simulink model "IM_Model"  (R2023a)
settings: Solver=ode23t  StartTime=0.0  StopTime=2  MaxStep=.0001  RelTol=1e-3
InitFcn:
  | Rs=0.5968;
  | Lls=0.0003495;
  | Rr=0.6258;
  | Llr=0.005473;
  | Lm=0.0354;
  | Ls=Lls+Lm;
  | Lr=Llr+Lm;
  | J=0.05;
  | B=0.005879;
  | P=4;
values from neighbouring files (symbols this model uses):
  Freq = 2*pi*50    (= 314.159265359)    [Parameters.m]
  Lms = Lm    (= 0.0353505)    [Parameters.m]
  Vin_Amp = 220*sqrt(2)    [Parameters.m]
libraries: spsControlledVoltageSourceLib x3, spsdq0toabcLib x2, spsAsynchronousMachineSIUnitsLib x1, spsabctodq0Lib x1, spspowerguiLib x1
settings Model: Creator=User  LastModifiedBy=User
settings DebuggingCC: UnconnectedInputMsg=warning  UnconnectedOutputMsg=warning  UnconnectedLineMsg=warning
settings ModelReferenceCC: EnableRefExpFcnMdlSchedulingChecks=on
settings RTWCC: DLArmComputeVersion=19.05

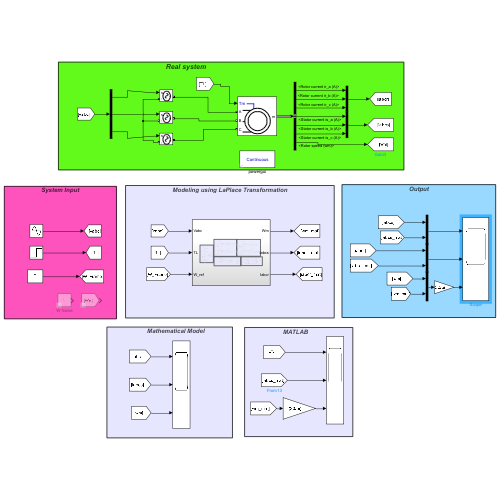
[thumbnail: Simulink's stored preview of the top-level diagram]
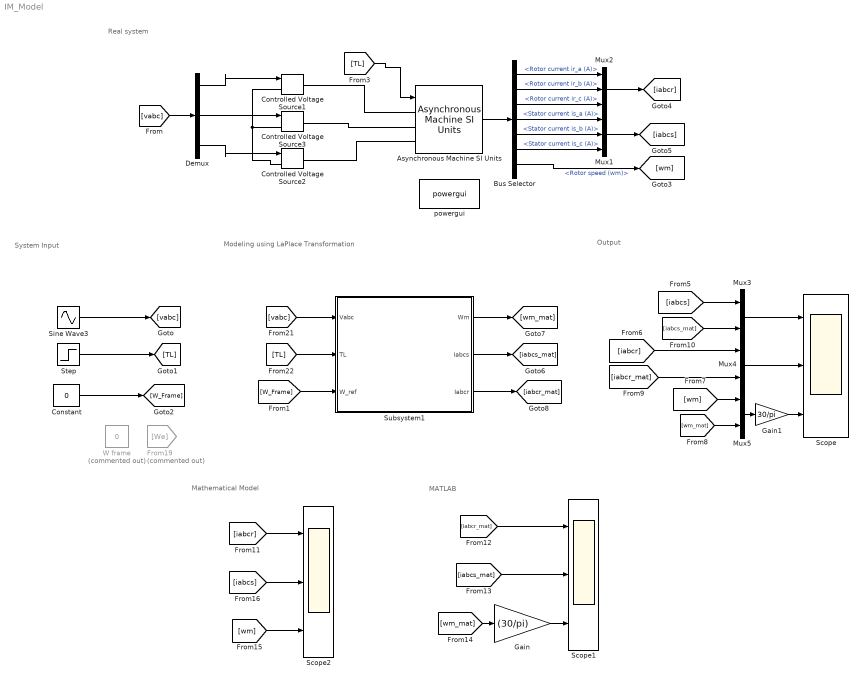
== system IM_Model ==
  note: Mathematical Model
  note: MATLAB
  note: Modeling using LaPlace Transformation
  note: Output
  note: System Input
  note: Real system
  Asynchronous Machine SI Units : spsAsynchronousMachineSIUnitsLib/Asynchronous Machine SI Units  RotorType=Squirrel-cage  PresetModel=No  MechanicalLoad=Torque Tm  ShowDetailedParameters=on  ReferenceFrame=Stationary  Units=SI  MeasurementBus=off  NominalParameters=[1e+04 400 50]  VoltageRatio=1  Stator=[Rs Lls]  Rotor=[Rr Llr]  Cage1=[0.4155 0.002066]  Cage2=[0.4168 0.0003495]  Lm=Lm  Mechanical=[J B P/2]  PolePairs=2  InitialConditions=[1 0 0 0 0 0 0 0]  SimulateSaturation=off  Saturation=[14.03593122, 27.81365428, 53.79336849, 72.68890987, 97.98006896, 148.6815601, 215.7428561, 302.9841135, 428.7778367 ; 230, 322, 414, 460, 506, 552, 598, 644, 690]  LoadFlowParameters=1492000  TsPowergui=0  TsBlock=-1  IterativeModel=Trapezoidal non iterative  IterativeDiscreteModel=Trapezoidal non iterative  Pmec=1.492e+006
  Bus Selector : BusSelector  OutputSignals=Rotor measurements.Rotor current ir_a (A),Rotor measurements.Rotor current ir_b (A),Rotor measurements.Rotor current ir_c (A),Stator measurements.Stator current is_a (A),Stator measurements.Stator current is_b (A),Stator measurements.Stator current is_c (A),Mechanical.Rotor speed (wm)
  Constant : Constant  Value=0
  Controlled Voltage Source1 : spsControlledVoltageSourceLib/Controlled Voltage Source  Initialize=on  Source_Type=AC  Amplitude=0  Phase=0  Frequency=0  Measurements=None
  Controlled Voltage Source2 : spsControlledVoltageSourceLib/Controlled Voltage Source  Initialize=on  Source_Type=AC  Amplitude=0  Phase=0  Frequency=0  Measurements=None
  Controlled Voltage Source3 : spsControlledVoltageSourceLib/Controlled Voltage Source  Initialize=on  Source_Type=AC  Amplitude=0  Phase=0  Frequency=0  Measurements=None
  Demux : Demux  Outputs=3
  From19 : From  Commented=on  GotoTag=We
  Gain : Gain  Gain=(30/pi)
  Gain1 : Gain  Gain=30/pi
  Mux1 : Mux  Inputs=3
  Mux2 : Mux  Inputs=3
  Mux3 : Mux  Inputs=2
  Mux4 : Mux  Inputs=2
  Mux5 : Mux  Inputs=2
  Scope : Scope  NumInputPorts=3
  Scope1 : Scope  NumInputPorts=3
  Scope2 : Scope  NumInputPorts=3
  Sine Wave3 : Sin  Amplitude=Vin_Amp  Frequency=Freq  Phase=[0 -2*pi/3 2*pi/3]  SampleTime=0
  Step : Step  Time=0  SampleTime=0
  Subsystem1 : Subsystem
  W frame : Constant  Commented=on  Value=0
  powergui : spspowerguiLib/powergui  Priority=1  SimulationMode=Continuous  SampleTime=50e-6  frequency=60  Iterations=50  frequencyindice=50  Pbase=100e6  ErrMax=1e-4  UnitsV=kV  UnitsW=MW  buscounter=0  FunctionMessages=off  echomessages=off  EnableUseOfTLC=off  CurrentSourceSwitches=off  DisableSnubberDevices=on  DisableRonSwitches=on  DisableVfSwitches=on  DisplayEquations=off  AutomaticDiscreteSolvers=off  SolverType=Tustin/Backward Euler (TBE)  Interpol=off  ExternalGateDelay=off  methode=off  Ts=100  x0status=blocks  SPID=on  SwTol=0  HookPort=off  NonlinearTolerance=1e-4  nMaxIteration=100  ContinueOnMaxIteration=off  RestoreLinks=warning  ResistiveCurrentMeasurement=off  Frange=[0:2:500]  Ylog=off  Xlog=on  ShowGrid=off  save=off  variable=ZData  structure=0  ZoomFFT=off  StartTime=0.0  cycles=1  DisplayStyle=1  fundamental=60  FreqAxis=off  MaxFrequency=1000  frequencyindicesteady=1  RmsSteady=1  display=off
  wires:
  Demux/1 -> Controlled Voltage Source1/1
  Demux/2 -> Controlled Voltage Source3/1
  Demux/3 -> Controlled Voltage Source2/1
  [vabc] -> Demux/1
  Sine Wave3/1 -> [vabc]
  Step/1 -> [TL]
  [TL] -> Asynchronous Machine SI Units/1
  Asynchronous Machine SI Units/1 -> Bus Selector/1
  Bus Selector/1 -> Mux2/1  "<Rotor current ir_a (A)>"
  Bus Selector/2 -> Mux2/2  "<Rotor current ir_b (A)>"
  Bus Selector/3 -> Mux2/3  "<Rotor current ir_c (A)>"
  Bus Selector/4 -> Mux1/1  "<Stator current is_a (A)>"
  Bus Selector/5 -> Mux1/2  "<Stator current is_b (A)>"
  Bus Selector/6 -> Mux1/3  "<Stator current is_c (A)>"
  Bus Selector/7 -> [wm]  "<Rotor speed (wm)>"
  Mux2/1 -> [iabcr]
  Mux1/1 -> [iabcs]
  [iabcs] -> Mux3/1
  [iabcs_mat] -> Mux3/2
  Mux3/1 -> Scope/1
  [iabcr_mat] -> Mux4/2
  [iabcr] -> Mux4/1
  Mux4/1 -> Scope/2
  [wm_mat] -> Mux5/2
  [wm] -> Mux5/1
  [iabcr_mat] -> Scope1/1
  [iabcs_mat] -> Scope1/2
  [wm_mat] -> Gain/1
  [iabcr] -> Scope2/1
  [wm] -> Scope2/3
  [iabcs] -> Scope2/2
  Constant/1 -> [W_Frame]
  Gain/1 -> Scope1/3
  [W_Frame] -> Subsystem1/3(W_ref)
  [TL] -> Subsystem1/2(TL)
  [vabc] -> Subsystem1/1(Vabc)
  Subsystem1/2(Iabcs) -> [iabcs_mat]
  Subsystem1/1(Wm) -> [wm_mat]
  Subsystem1/3(Iabcr) -> [iabcr_mat]
  Mux5/1 -> Gain1/1
  Gain1/1 -> Scope/3
  connections:
  Controlled Voltage Source2/LConn1 -- Controlled Voltage Source1/LConn1 -- Controlled Voltage Source3/LConn1
  Controlled Voltage Source1/RConn1 -- Asynchronous Machine SI Units/LConn1
  Controlled Voltage Source3/RConn1 -- Asynchronous Machine SI Units/LConn2
  Controlled Voltage Source2/RConn1 -- Asynchronous Machine SI Units/LConn3

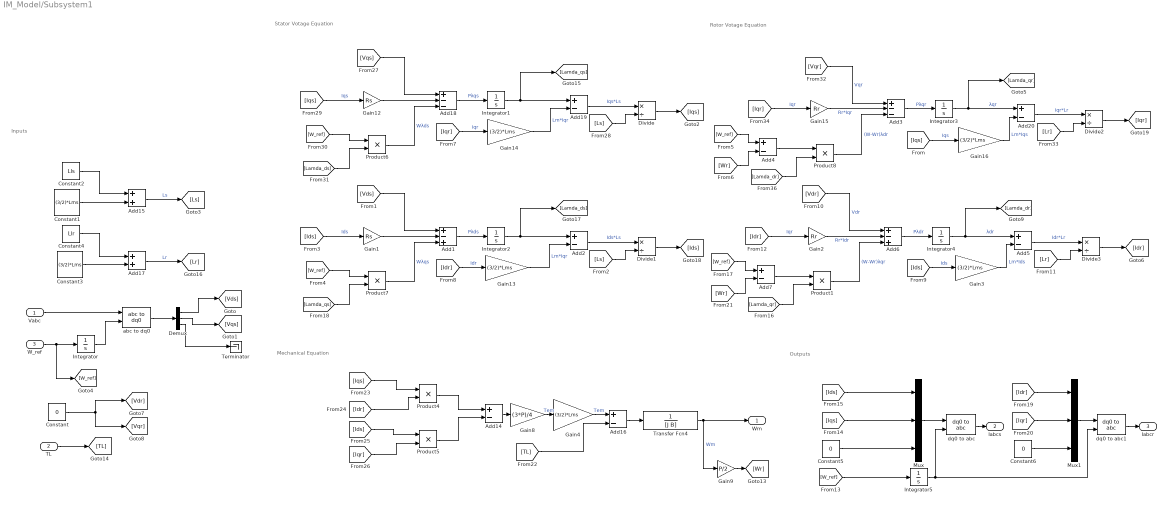
== system IM_Model/Subsystem1 ==
  note: Outputs
  note: Rotor Votage Equation
  note: Stator Votage Equation
  note: Mechanical Equation
  note: Inputs
  Vabc : Inport
  TL : Inport  Port=2
  W_ref : Inport  Port=3
  Add1 : Sum  Inputs=+-+
  Add{2,4..5,7,14,16,19..20} (8 alike) : Sum  Inputs=+-
  Add15 : Sum
  Add17 : Sum
  Add18 : Sum  Inputs=+--
  Add3 : Sum  Inputs=+--
  Add6 : Sum  Inputs=+-+
  Constant : Constant  Value=0
  Constant1 : Constant  Value=(3/2)*Lms
  Constant2 : Constant  Value=Lls
  Constant3 : Constant  Value=(3/2)*Lms
  Constant4 : Constant  Value=Llr
  Constant5 : Constant  Value=0
  Constant6 : Constant  Value=0
  Demux : Demux  Outputs=3
  Divide{,1..3} (4 alike) : Product  Inputs=*/
  Gain1 : Gain  Gain=Rs
  Gain12 : Gain  Gain=Rs
  Gain{3..4,13..14,16} (5 alike) : Gain  Gain=(3/2)*Lms
  Gain15 : Gain  Gain=Rr
  Gain2 : Gain  Gain=Rr
  Gain8 : Gain  Gain=(3*P)/4
  Gain9 : Gain  Gain=P/2
  Integrator{,1..5} (6 alike) : Integrator
  Mux : Mux  Inputs=3
  Mux1 : Mux  Inputs=3
  Product{1,4..8} (6 alike) : Product
  Terminator : Terminator
  Transfer Fcn4 : TransferFcn  Denominator=[J B]
  abc to dq0 : spsabctodq0Lib/abc to dq0  Alignment=Aligned with phase A axis
  dq0 to abc : spsdq0toabcLib/dq0 to abc  Alignment=90 degrees behind phase A axis
  dq0 to abc1 : spsdq0toabcLib/dq0 to abc  Alignment=90 degrees behind phase A axis
  Wm : Outport
  Iabcs : Outport  Port=2
  Iabcr : Outport  Port=3
  wires:
  Gain9/1 -> [Wr]
  Transfer Fcn4/1 -> Wm/1, Gain9/1  "Wm"
  Add16/1 -> Transfer Fcn4/1
  [TL] -> Add16/2
  Gain8/1 -> Gain4/1  "Tem"
  Add14/1 -> Gain8/1
  Product5/1 -> Add14/2
  Product4/1 -> Add14/1
  [Iqr] -> Product5/2
  [Ids] -> Product5/1
  [Idr] -> Product4/2
  [Iqs] -> Product4/1
  TL/1 -> [TL]
  Constant/1 -> [Vqr], [Vdr]
  Demux/3 -> Terminator/1
  Demux/2 -> [Vqs]
  Demux/1 -> [Vds]
  abc to dq0/1 -> Demux/1
  Integrator/1 -> abc to dq0/2
  W_ref/1 -> Integrator/1, [W_ref]
  Vabc/1 -> abc to dq0/1
  Product6/1 -> Add18/3  "Wλds"
  [W_ref] -> Product6/1
  [Lamda_ds] -> Product6/2
  [Vqs] -> Add18/1
  Gain12/1 -> Add18/2
  [Iqs] -> Gain12/1  "Iqs"
  Add18/1 -> Integrator1/1  "Pλqs"
  Integrator1/1 -> Add19/1, [Lamda_qs]
  Constant1/1 -> Add15/2
  Constant2/1 -> Add15/1
  Add15/1 -> [Ls]  "Ls"
  Add17/1 -> [Lr]  "Lr"
  Constant4/1 -> Add17/1
  Constant3/1 -> Add17/2
  Gain14/1 -> Add19/2  "Lm*Iqr"
  [Iqr] -> Gain14/1  "Iqr"
  Add19/1 -> Divide/1  "Iqs*Ls"
  [Ls] -> Divide/2
  Divide/1 -> [Iqs]
  Divide1/1 -> [Ids]
  [Ls] -> Divide1/2
  Add2/1 -> Divide1/1  "Ids*Ls"
  [Idr] -> Gain13/1  "Idr"
  Gain13/1 -> Add2/2  "Lm*Iqr"
  Integrator2/1 -> [Lamda_ds], Add2/1
  Add1/1 -> Integrator2/1  "Pλds"
  [Ids] -> Gain1/1  "Ids"
  Gain1/1 -> Add1/2
  [Vds] -> Add1/1
  [Lamda_qs] -> Product7/2
  [W_ref] -> Product7/1
  Product7/1 -> Add1/3  "Wλqs"
  Divide2/1 -> [Iqr]
  [Lr] -> Divide2/2
  Add20/1 -> Divide2/1  "Iqr*Lr"
  [Iqs] -> Gain16/1  "Iqs"
  Gain16/1 -> Add20/2  "Lm*Iqs"
  Integrator3/1 -> [Lamda_qr], Add20/1  "λqr"
  Add3/1 -> Integrator3/1  "Pλqr"
  [Iqr] -> Gain15/1  "Iqr"
  Gain15/1 -> Add3/2  "Rr*Iqr"
  [Vqr] -> Add3/1  "Vqr"
  [Lamda_dr] -> Product8/2
  Product8/1 -> Add3/3  "(W-Wr)λdr"
  [W_ref] -> Add4/1
  [Wr] -> Add4/2
  Add4/1 -> Product8/1
  Add7/1 -> Product1/1
  [Wr] -> Add7/2
  [W_ref] -> Add7/1
  Product1/1 -> Add6/3  "(W-Wr)λqr"
  [Lamda_qr] -> Product1/2
  [Vdr] -> Add6/1  "Vdr"
  Gain2/1 -> Add6/2  "Rr*Idr"
  [Idr] -> Gain2/1  "Iqr"
  Add6/1 -> Integrator4/1  "Pλdr"
  Integrator4/1 -> Add5/1, [Lamda_dr]  "λdr"
  Gain3/1 -> Add5/2  "Lm*Ids"
  [Ids] -> Gain3/1  "Ids"
  Add5/1 -> Divide3/1  "Idr*Lr"
  [Lr] -> Divide3/2
  Divide3/1 -> [Idr]
  [W_ref] -> Integrator5/1
  [Iqs] -> Mux/2
  [Ids] -> Mux/1
  Constant5/1 -> Mux/3
  Mux/1 -> dq0 to abc/1
  dq0 to abc/1 -> Iabcs/1
  Gain4/1 -> Add16/1  "Tem"
  [Iqr] -> Mux1/2
  [Idr] -> Mux1/1
  Constant6/1 -> Mux1/3
  Mux1/1 -> dq0 to abc1/1
  Integrator5/1 -> dq0 to abc/2, dq0 to abc1/2
  dq0 to abc1/1 -> Iabcr/1
